simulink model "CrazyPendrum"  (R2014a)
settings: Solver=ode45  StartTime=0.0  StopTime=10.0  RelTol=1e-3
libraries: vrlib x2
settings Model: Creator=Anton  LastModifiedBy=hollowman
settings DebuggingCC: UnderspecifiedInitializationDetection=Classic

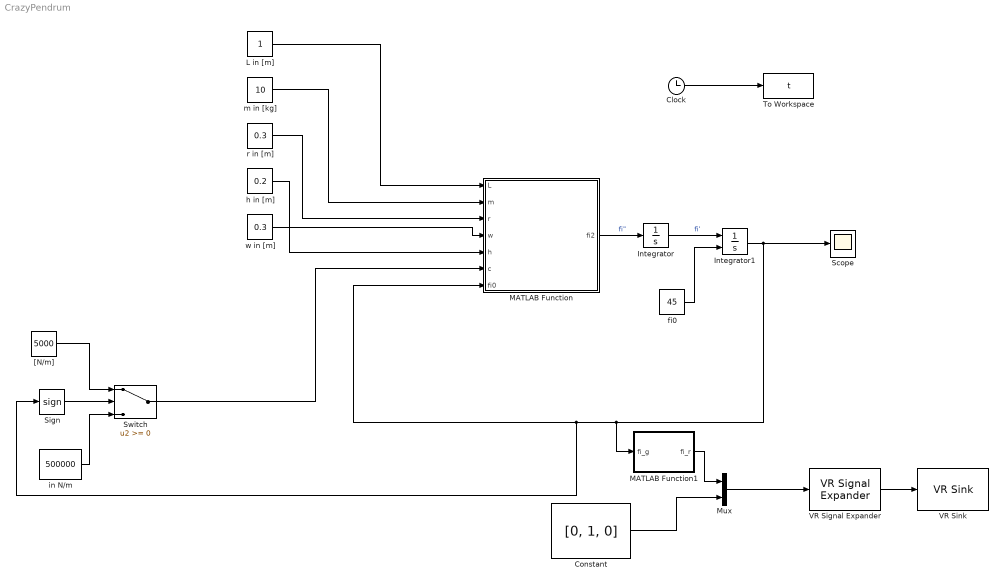
== system CrazyPendrum ==
  Clock : Clock
  Constant : Constant  Value=[0, 1, 0]
  Integrator : Integrator
  Integrator1 : Integrator  InitialConditionSource=external
  L in [m] : Constant
  MATLAB Function : MATLAB Function  TreatAsAtomicUnit=on
  MATLAB Function1 : MATLAB Function  TreatAsAtomicUnit=on
  Mux : Mux  Inputs=2
  Scope : Scope
  Sign : Signum
  Switch : Switch
  To Workspace : ToWorkspace  VariableName=t  SampleTime=-1
  VR Signal Expander : vrlib/VR Signal Expander  outwidth=4  outidx=[4 1 2 3]
  VR Sink : vrlib/VR Sink  InstantiateOnLoad=on  SampleTime=0.005  ViewEnable=on  RemoteChange=off  RemoteView=off  FieldsWritten=Seiltrommel.rotation.4.1.1.double  WorldFileName=CrazyPendlm.wrl  AutoView=off  VideoDimensions=[]  AllowVariableSize=off
  "[N/m]" : Constant  Value=5000
  fi0 : Constant  Value=45
  h in [m] : Constant  Value=0.2
  in N/m : Constant  Value=500000
  m in [kg] : Constant  Value=10
  r in [m] : Constant  Value=0.3
  w in [m] : Constant  Value=0.3
  wires:
  Sign/1 -> Switch/2
  "[N/m]"/1 -> Switch/1
  in N/m/1 -> Switch/3
  Integrator1/1 -> MATLAB Function1/1(fi_g), MATLAB Function/7(fi0), Sign/1, Scope/1
  Integrator/1 -> Integrator1/1  "fi'"
  Switch/1 -> MATLAB Function/6(c)
  L in [m]/1 -> MATLAB Function/1(L)
  m in [kg]/1 -> MATLAB Function/2(m)
  r in [m]/1 -> MATLAB Function/3(r)
  h in [m]/1 -> MATLAB Function/5(h)
  w in [m]/1 -> MATLAB Function/4(w)
  fi0/1 -> Integrator1/2
  MATLAB Function/1(fi2) -> Integrator/1  "fi\""
  Constant/1 -> Mux/2
  Mux/1 -> VR Signal Expander/1
  MATLAB Function1/1(fi_r) -> Mux/1
  Clock/1 -> To Workspace/1
  VR Signal Expander/1 -> VR Sink/1

== matlab function CrazyPendrum/MATLAB Function1 ==
  data: fi_g input; fi_r output
function fi_r = fcn(fi_g)
%#codegen

fi_r = fi_g * pi() / 180;

== matlab function CrazyPendrum/MATLAB Function ==
  data: L input; fi2 output; m input; r input; w input; h input; c input; fi0 input
function fi2 = fcn(L,m,r,w,h,c,fi0)

g = 9.81; %
Fg = g * m;

M_t = Fg * cos(fi0) * (L+h/2);
M_f = (c*(fi0*pi()/180) * r)*r;

J_a = m/12 * (w^2+h^2)+m*(L+h/2)^2;

fi2 = (M_t-M_f)/J_a;
